simulink model "pidreg"  (R2021b)
settings: Solver=VariableStepAuto  StartTime=0.0  StopTime=10.0  RelTol=1e-3
undefined symbols (not defined in the file): Angle, J, Kd, ke, Ki, km, Kp, L, Moth, R
settings Model: Creator=vital  LastModifiedBy=vital
settings SolverCC: AlgebraicLoopSolver=TrustRegion
settings DebuggingCC: SFMachineParentedDataDiag=warning

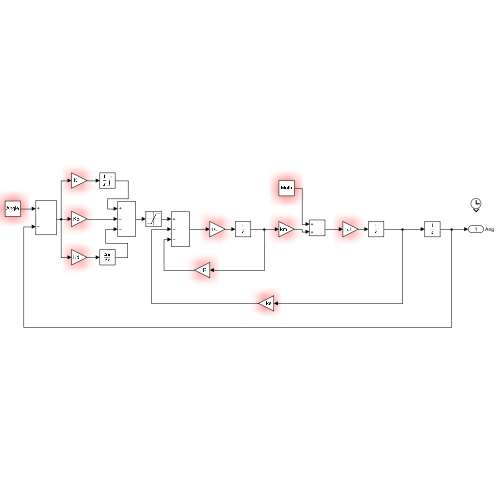
[thumbnail: Simulink's stored preview of the top-level diagram]
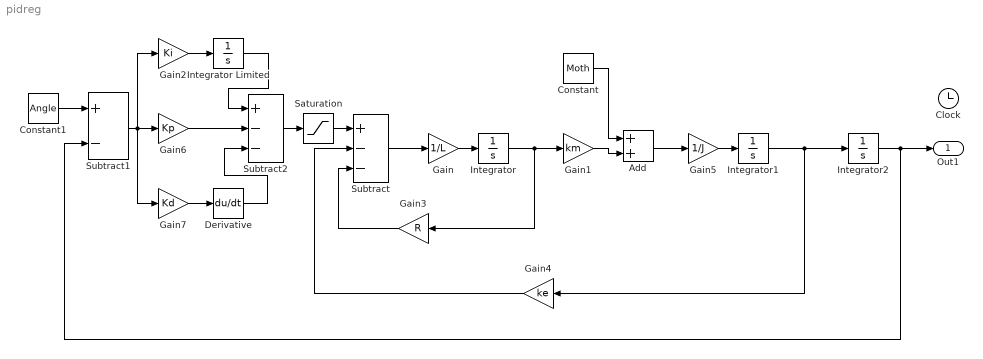
== system pidreg ==
  Add : Sum
  Clock : Clock
  Constant : Constant  Value=Moth
  Constant1 : Constant  Value=Angle
  Derivative : Derivative
  Gain : Gain  Gain=1/L
  Gain1 : Gain  Gain=km
  Gain2 : Gain  Gain=Ki
  Gain3 : Gain  Gain=R
  Gain4 : Gain  Gain=ke
  Gain5 : Gain  Gain=1/J
  Gain6 : Gain  Gain=Kp
  Gain7 : Gain  Gain=Kd
  Integrator : Integrator
  Integrator Limited : Integrator  LimitOutput=on  UpperSaturationLimit=2  LowerSaturationLimit=0
  Integrator1 : Integrator
  Integrator2 : Integrator
  Saturation : Saturate  UpperLimit=6.87  LowerLimit=-6.87
  Subtract : Sum  Inputs=+--
  Subtract1 : Sum  Inputs=+-
  Subtract2 : Sum  Inputs=+--
  Out1 : Outport  SignalName=Ang
  wires:
  Subtract/1 -> Gain/1
  Gain/1 -> Integrator/1
  Constant1/1 -> Subtract1/1
  Subtract1/1 -> Gain7/1, Gain2/1, Gain6/1
  Saturation/1 -> Subtract/1
  Integrator/1 -> Gain3/1, Gain1/1
  Gain3/1 -> Subtract/3
  Gain4/1 -> Subtract/2
  Integrator1/1 -> Gain4/1, Integrator2/1
  Integrator2/1 -> Subtract1/2, Out1/1
  Gain5/1 -> Integrator1/1
  Gain1/1 -> Add/2
  Add/1 -> Gain5/1
  Constant/1 -> Add/1
  Gain2/1 -> Integrator Limited/1
  Gain7/1 -> Derivative/1
  Subtract2/1 -> Saturation/1
  Gain6/1 -> Subtract2/2
  Derivative/1 -> Subtract2/3
  Integrator Limited/1 -> Subtract2/1
